simulink library "rtlsdr_book_library"  (R2014b)
settings: Solver=ode45  StartTime=0.0  StopTime=10.0  RelTol=1e-3
values from neighbouring files (symbols this model uses):
  frm = rmfield(frm , 'master_frame')    [image_frame_gen.m]    (also in import_rtlsdr_data.m = cast(frm,obj.data_type))
  src = rmfield(src , 'master_time')    [ASCII_frame_gen.m]
undefined symbols (not defined in the file or in its folder): den, dfilt, fdesignblkfcn, gcbh, iir, num, rtlsdr_frmsize, rtlsdr_fs
undefined symbols (not defined in the file): costas
libraries: dspsigops x6, commsynccomp2 x4, dspsrcs4 x2, dspstat3 x2, dspobslib x2, simulink_extras x2, dspmtrx3 x2, dsparch4 x1, rtlsdr_book_library x1, dspspect3 x1, commrflib2 x1
(part 1 of 5)
Description:
  | Software, Simulation Examples and Design Exercises Licence Agreement
  | 
  | This license agreement refers to the simulation examples, design exercises and files,
  | and associated software MATLAB and Simulink resources that accompany the book:
  | 
  |      Title: Software Defined Radio using MATLAB & Simulink and the RTL-SDR
  |      Published by Strathclyde Academic Media, 2015
  |      Authored by Robert W. Stewart, Kenneth W. Barlee, Dale S.W. Atkinson,
  |      and Louise H. Crockett
  | 
  | and made available as a download from, www.desktopSDR.com or variously acquired
  | by other means such as via USB storage, cloud storage, disk or any other electronic
  | or optical or magnetic storage mechanism. These files and associated software may
  | be used subject to the terms of agreement of the conditions below:
  | 
  |     Copyright © 2015 Robert W. Stewart, Kenneth W. Barlee, Dale S.W. Atkinson,
  |     and Louise H. Crockett
  |     All rights reserved.
  | 
  | Redistribution and use in source and binary forms, with or without modification, are
  | permitted provided that the following conditions are met:
  | 
  |    1.  Redistributions of source code must retain the above copyright notice, this list of
  |         conditions and the following disclaimer.
  | 
  |    2.  Redistributions in binary form must reproduce the above copyright notice, this
  |         list of conditions and the following disclaimer in the documentation and/or other
  |         materials provided with the distribution.
  | 
  |    3.  Neither the name of the copyright holder nor the names of its contributors may
  |         be used to endorse or promote products derived from this software without
  |         specific prior written permission.
  | 
  |    4.  In all cases, the software is, and all modifications and derivatives of the
  |         software shall be, licensed to you solely for use in conjunction with The
  |         MathWorks, Inc. products and service offerings.
  | 
  | THIS SOFTWARE IS PROVIDED BY THE COPYRIGHT HOLDERS AND CONTRIBUTORS
  | "AS IS" AND ANY EXPRESS OR IMPLIED WARRANTIES, INCLUDING, BUT NOT LIMITED
  | TO, THE IMPLIED WARRANTIES OF MERCHANTABILITY AND FITNESS FOR A
  | PARTICULAR PURPOSE ARE DISCLAIMED. IN NO EVENT SHALL THE COPYRIGHT
  | HOLDER OR CONTRIBUTORS BE LIABLE FOR ANY DIRECT, INDIRECT, INCIDENTAL,
  | SPECIAL, EXEMPLARY, OR CONSEQUENTIAL DAMAGES (INCLUDING, BUT NOT
  | LIMITED TO, PROCUREMENT OF SUBSTITUTE GOODS OR SERVICES; LOSS OF USE,
  | DATA, OR PROFITS; OR BUSINESS INTERRUPTION) HOWEVER CAUSED AND ON ANY
  | THEORY OF LIABILITY, WHETHER IN CONTRACT, STRICT LIABILITY, OR TORT
  | (INCLUDING NEGLIGENCE OR OTHERWISE) ARISING IN ANY WAY OUT OF THE USE
  | OF THIS SOFTWARE, EVEN IF ADVISED OF THE POSSIBILITY OF SUCH DAMAGE.
  | 
  | 
  | Audio Tracks used in Simulations Examples and Design Exercises
  | 
  | The music and vocal files used within the Examples files and software within the book
  | were variously written, arranged, performed, recorded and produced by Garrey Rice,
  | Adam Struth, Jamie Struth, Iain Thistlethwaite and also Marshall Craigmyle who
  | collectively, and individually where appropriate, assert and retain all of their copyright,
  | performance and artistic rights. Permission to use and reproduce this music is
  | granted for all purposes associated with MATLAB and Simulink software and the
  | simulation examples and design exercises files that accompany this book. Requests to
  | use the music for any other purpose should be directed to: info@desktopSDR.com.
  | For information on music track names, full credits, and links to the musicians please
  | refer to www.desktopSDR.com/more/audio.
settings Model: Creator=dkb10130  LastModifiedBy=ehb10152

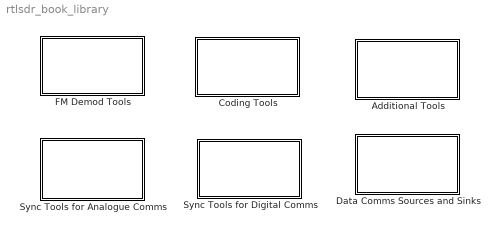
== system rtlsdr_book_library ==
  Additional Tools : Subsystem
      mask Display: disp('Additional\nTools');
  Coding Tools : Subsystem
      mask Display:
      | plot(-2,-2.5,...
      |      105,1.1,...
      |      [0  10 10.1 50 50.1 60 60.01 100],[0 0 1 1 0 0 1 1]); % bitstream
      | 
      | disp('\nCoding\nTools ');
  Data Comms Sources and Sinks : Subsystem
      mask Display:
      | plot(-2,-2.5,...
      |      105,1.1,...
      |      [45 45.01 50 50.01 55 55.01 60 60.01 65 65.01 70 70.01 75 75.01 80 80.01 85 85.01 90 90.01 95 95.01 100],...
      |      [0  1    1  0    0  0    0  1    1  0    0  1    1  1    1  0     0  1    1  0     0  1    1]); % bitstream
      | 
      | disp('\n010110                 \n\n\n\n')
      | disp('\nData Sources\nand Sinks');
  FM Demod Tools : Subsystem
      mask Display:
      | i = sin(2*pi*12*[0:0.001:0.4]);
      | fm = 2*sin(2*pi*80*[0:0.001:0.4] + cumsum(i)/3);
      | 
      | plot(-0.01,-13,...
      |     0.41,2.5,...
      |     [0:0.001:0.4], [fm(21:219), -2.5, 2.5, 2*i(202:end)]);
      | 
      | clear('i','fm');
      | 
      | disp('\nFM Demod\nTools');
  Sync Tools for Analogue Comms : Subsystem
      mask Display:
      | i = sin(2*pi*12*[0:0.001:0.4]);
      | am = sin(2*pi*99*[0:0.001:0.4]) .* (i+1.5);
      | 
      | plot(-0.01,-13,...
      |     0.41,2.5,...
      |     [0:0.001:0.4], [am(21:219), -2.5, 2.5, 2*i(202:end)]);
      | 
      | clear('i','am');
      | 
      | disp('\nSync Tools for\nAnalogue Comms');
  Sync Tools for Digital Comms : Subsystem
      mask Display:
      | plot(-2,-2.5,...
      |      125,1.1,...
      |      [5 15 15.1 30 30 45 45.1 60 60.1 75 75.1 90 90.1 105 105.1 115],[0.5 0.5 1 1 0.2 0.2 1 1 0.2 0.2 1 1 0.2 0.2 0.5 0.5]);  % Received Signal
      | 
      | plot(-2,-2.5,...
      |      125,1.1,...
      |      [5 11.5 11.6 27 27 42.5 42.6 58 58.1 73.5 73.6 89 89.1 104.5 104.6 115],[0.3,0.3,0.8,0.8,-0.1,-0.1,0.8,0.8,-0.1,-0.1,0.8,0.8,-0.1,-0.1,0.3,0.3]);  % Local Signal
      | 
      | disp('\nSync Tools for\nDigital Comms');

== system rtlsdr_book_library/Additional Tools ==
  433MHz Tuner Freq and Gain Control : Subsystem  mask{tuner_freq=433.0, tuner_gain=25}
      mask prompts: tuner_freq "Frequency (MHz)"; tuner_gain "Gain (dB)"
      mask DialogControl DescGroupVar Prompt: Tuner Frequency and Gain Control
      mask DialogControl DescTextVar Prompt: Use the control below to change the tuner frequency and gain.
  AM-SSB Modulator : Subsystem  mask{ac=1, phc=0, fc=40e3, fs=120e3, frm_size=1500}
      mask prompts: ac "Carrier Amplitude:"; phc "Carrier Phase (rads):"; fc "Carrier Frequency (Hz):"; fs "Sampling Frequency (Hz):"; frm_size "Output Frame Size:"
      mask DialogControl DescTextVar Prompt: This block AM-SSB modulates an information signal, outputting both the AM-SLSB and AM-SUSB variants. We have also output the carrier, which can be used as a reference.
  Import RTL-SDR Data : Subsystem  InitFcn=|  StopFcn=|  mask{filename=rtlsdr_data.mat, frm_size=4096, data_type=single}
      InitFcn=|
      | try
      |    load(get_param(gcb,'filename'));
      |    [nfrm,rtlsdr_frmsize] = size(rtlsdr_data.data);
      |    rtlsdr_fs = rtlsdr_frmsize/rtlsdr_data.TimeInfo.Increment;
      | catch
      |       error(['Unable to read file "',get_param(gcbh,'filename'),...
      |            '". No such file or directory. Please check that the filename',...
      |            ' you entered is correct, and contains the ".mat" extension.']);
      | end
      StopFcn=|
      | clear(...
      | 'rtlsdr_frmsize',...
      | 'rtlsdr_fs',...
      | 'nfrm',...
      | 'rtlsdr_data' );
      mask prompts: filename "File Name:"; frm_size "Output Frame Size:"; data_type "Output Data Type:"
      settings: CloseFcn=|
      | try
      |    load(get_param(gcb,'filename'));
      |    [nfrm,rtlsdr_frmsize] = size(rtlsdr_data.data);
      |    rtlsdr_fs = rtlsdr_frmsize/rtlsdr_data.TimeInfo.Increment;
      | catch
      |       error(['Unable to read file "',get_param(gcbh,'filename'),...
      |            '". No such file or directory. Please check that the filename',...
      |            ' you entered is correct, and contains the ".mat" extension.']);
      | end
      mask Callback filename:
      | set_param([gcb '/From File'], 'Filename',...
      |             get_param(gcbh,'filename'));
      mask TypeOptions data_type: int16 | single | double
      mask DialogControl Control2 Prompt: Browse
      mask DialogControl Control2 Callback:
      | % browse for file
      | [filename,path] = uigetfile({'*.mat'},'Select an RTL-SDR Data File');
      | 
      | % if in current folder, only use filename
      | if strcmp([pwd,filesep],path)
      | 
      |     try
      |         % try to set the filename in the box
      |         set_param(...
      |             gcb,...
      |             'filename',...
      |             filename );
      |         % try to import the data
      |         load(get_param(gcb,'filename'));
      |         rtlsdr_frmsize = length(rtlsdr_data.data);
      |         [nfrm,rtlsdr_frmsize] = size(rtlsdr_data.data);
      |         rtlsdr_fs = rtlsdr_frmsize/rtlsdr_data.TimeInfo.Increment;
      |     end
      | % else use full filepath
      | else
      | 
      |     try
      |         % try to set the filename in the box
      |         set_param(...
      |             gcb,...
      |             'filename',...
      |             [path,filename] );
      |         % try to import the data
      |      	load(get_param(gcb,'filename'));
      |         [nfrm,rtlsdr_frmsize] = size(rtlsdr_data.data);
      |         rtlsdr_fs = rtlsdr_frmsize/rtlsdr_data.TimeInfo.Increment;
      |     end
      | end
      | 
      | clear('path','filename');
      mask Display:
      | % try to apply icon
      | try
      |     root = which('rtlsdr_book_library');
      |     root = root(1:end-length('rtlsdr_book_library/rtlsdr_book_library.slx'));
      |     image([root,'rtlsdr_book_library/block_icons/icon__load_rtlsdr_data.png'],[0,0,125,60]);
      | end
      | 
      | % if file accessible
      | try
      |     load(get_param(gcb,'filename'));
      |         [nfrm,rtlsdr_frmsize] = size(rtlsdr_data.data);
      |         rtlsdr_fs = rtlsdr_frmsize/rtlsdr_data.TimeInfo.Increment;
      |         %rtlsdr_fs = 1/rtlsdr_data.TimeInfo.Increment;
      | 
      |     % convert to kHz
      |     fs = rtlsdr_fs/1000;
      | 
      |     % if MHz.. convert to MHz and display
      |     if fs > 999
      |         fs = fs/1000;
      |         fprintf(['\n\n\n               fs = ',num2str(fs),'MHz']);
      | 
      |     % else display kHz
      |     else
      |         fprintf(['\n\n\n              fs = ',num2str(fs),'kHz']);
      |     end
      | 
      | catch
      |     % display nothing
      |     fprintf('\n\n\n   fs = ');
      | end
  Model Information : Subsystem
  Remove DC Component : Subsystem
      mask DialogControl DescGroupVar Prompt: Remove DC Component
      mask DialogControl DescTextVar Prompt: This block removes the DC component of signals input to it.
  Save RTL-SDR Data : Subsystem  InitFcn=|  mask{file_name=rtlsdr_data.mat}
      | stop_time = get_param(gcs,'StopTime');
      | 
      | if str2num(stop_time) > 120
      | 
      |    dlg = warndlg(...
      |       ['Running this simulation for ',stop_time,' seconds will create a very large data file!'],...
      |       'Warning: Save RTL-SDR Data',...
      |       'modal');
      |    
      |    uiwait(dlg);
      | 
      | end
      | 
      | clear('stop_time');
      mask prompts: file_name "File Name:"
      mask Callback file_name:
      | set_param([gcb '/To File'], 'Filename',...
      |             get_param(gcbh,'file_name'))
      mask DialogControl Control3 Prompt: Browse
      mask DialogControl Control3 Callback:
      | % browse for file
      | [filename,path] = uiputfile({'*.mat'},'Create an RTL-SDR Data File');
      | 
      | % if in current folder, only use filename
      | if strcmp([pwd,filesep],path)
      | 
      |     % try to set the filename in the box
      |     try
      |         set_param(...
      |             gcb,...
      |             'file_name',...
      |             filename );
      |     end
      | % else use full filepath
      | else
      | 
      |     % try to set the filename in the box
      |     try
      |         set_param(...
      |             gcb,...
      |             'file_name',...
      |             [path,filename] );
      |     end
      | end
      | 
      | clear('path','filename');
      mask Display:
      | % try to apply icon
      | try
      |     root = which('rtlsdr_book_library');
      |     root = root(1:end-length('rtlsdr_book_library/rtlsdr_book_library.slx'));
      |     image([root,'rtlsdr_book_library/block_icons/icon__save_rtlsdr_data.png'],[0,0,125,60]);
      | end

== system rtlsdr_book_library/Coding Tools ==
  Differential QPSK Decoder : Subsystem  mask{op_buff_len=2}
      mask prompts: op_buff_len "Enter the required output frame size:"
      mask DialogControl DescGroupVar Prompt: Differential QPSK Decoder
      mask DialogControl DescTextVar Prompt: This subsystem contains the combinatorial logic required to implement a QPSK Decoder.
  Differential QPSK Encoder : Subsystem  mask{op_buff_len=2}
      mask prompts: op_buff_len "Enter the required output frame size:"
      mask DialogControl DescGroupVar Prompt: Differential QPSK Encoder
      mask DialogControl DescTextVar Prompt: This subsystem contains the combinatorial logic required to implement a QPSK Encoder.

== system rtlsdr_book_library/Data Comms Sources and Sinks ==
  "  ASCII Transfer Binary Source" : Subsystem  mask(Bit Source Generator - Numbered Frames){msg_tx=Hello World!, fs=2e3, ascii_len=8}
      mask prompts: msg_tx "Message String:"; fs "Bitrate (Sampling Frequency):"; ascii_len "ASCII Character Bit Length:"
      mask help: The block converts ASCII characters from the 'Message String' field to ASCII bits. This then forms the payload of an individual frame and is appended to the preamble sequence, which forms the header. The output of this block is a data frame of bits that will be modulated and transmitted.
      mask init:
      | try
      |     ASCII_frame_gen;
      | catch ME
      |     if(strcmp(ME.identifier,'MATLAB:UndefinedFunction'))
      |         error('Unable to find "ASCII_frame_gen.m".');
      |     end
      |     rethrow(ME);
      | end
      settings: ModelCloseFcn=clear('msg_output','rec','run_time','src')
      mask Callback msg_tx: ASCII_frame_gen;
      mask Callback fs: ASCII_frame_gen;
      mask Callback ascii_len: ASCII_frame_gen;
      mask Display:
      | try
      |     ASCII_frame_gen;
      | catch ME
      |     if(strcmp(ME.identifier,'MATLAB:UndefinedFunction'))
      |         error('Unable to find "ASCII_frame_gen.m".');
      |     end
      |     rethrow(ME);
      | end
      | 
      | %% FOR MASK
      | % number of chars in message
      | src.num_chars = src.len(:,1);
      | % create text string
      | icon_text = ['Bit Source - Numbered Frames\n\n'...
      |              'Message Length (chars) = ',num2str(src.num_chars),'\n\n'...
      |              'Frame Size (bits) = ',num2str(src.master_frame_len)];
      | % display on block
      | disp(icon_text);
  ASCII Decoding : Subsystem  mask(ASCII Reconstruction){msg_len=16, ascii_len=8}
      mask prompts: msg_len "Message Length (chars):"; ascii_len "ASCII Character Bit Length:"
      mask help: The block reconstructs the ASCII strings from the input payload.
  Image Reconstruction : Subsystem  InitFcn=|  mask(Image Reconstruction){}
      | % create figure window, plot empty image then hide
      | hfig = figure;
      | imshow(uint8(zeros(100,100)),'InitialMagnification',250);
      | hfig.Visible = 'off';
      mask help: This block will receive and process frames of image data. When the full image has been receieved, the simulation will pause, and the image will be displayed.
      settings: CloseFcn=clear('hfig','hax');
      settings: PauseFcn=|
      | % set current figure to handle
      | set(0,'CurrentFigure',hfig);
      | 
      | % make plot visible if not already
      | hfig.Visible = 'on'
      | 
      | % plot image
      | imshow(uint8(image),'InitialMagnification',250);
      | 
      | % configure image figure window
      | hfig.MenuBar = 'none';
      | hfig.ToolBar = 'none';
      | hfig.Resize = 'off';
      | hfig.Name = 'Received Image';
      | hfig.NumberTitle = 'off';
      | hfig.Position = [hfig.Position(1)+45,hfig.Position(2)+3,330,335];
      | hax = gca;
      | hax.Units = 'pixels';
      | hax.Position = [40,45,250,250];
      | 
      | % resume simulation
      | set_param(bdroot, 'SimulationCommand', 'continue')
  Image Transfer Binary Source : Subsystem  mask(Bit Source Generator - Image Transfer){filename=image1.mat, fs=2e3, binary_len=8}
      mask prompts: filename "Image Filename:"; fs "Bitrate (Sampling Frequency):"; binary_len "Image Pixel Bit Depth:"
      mask help: The block allows the user to enter the filename of an image that they wish to transmit. It converts the image's pixels from decimal values to binary bit representations, and generates the number of frames required to transfer the data to the receiver. Each frame's header has a preamble and a number of fields that contain information about the frame, to support the recovery of the data at the receiver. The remaining space in each frame is then dedicated to the payload, which contains a part of the total data to be transferred.
      mask init:
      | try
      |     image_frame_gen;
      | catch ME
      |     switch ME.identifier
      |         case 'MATLAB:load:couldNotReadFile'
      |             error(['Unable to locate "', get_param(gcb,'filename'),'". Please check that the image filename is correct.']);
      |         case 'MATLAB:UndefinedFunction'
      |             error('Unable to find "image_frame_gen.m".');
      |         otherwise
      |             rethrow(ME)
      |     end
      | end
      settings: ModelCloseFcn=clear('frm')
      mask Callback filename:
      | %% PULL DATA FROM MASK
      | frm.filename = get_param(gcbh,'filename');
      | 
      | set_param(gcb,'filename',frm.filename)
      | 
      | try
      |     image_frame_gen;
      | catch ME
      |     switch ME.identifier
      |         case 'MATLAB:load:couldNotReadFile'
      |             error(['Unable to locate "', get_param(gcb,'filename'),'". Please check that the image filename is correct.']);
      |         case 'MATLAB:UndefinedFunction'
      |             error('Unable to find "image_frame_gen.m".');
      |         otherwise
      |             rethrow(ME)
      |     end
      | end
      mask Callback fs:
      | %% PULL DATA FROM MASK
      | frm.fs = str2num(get_param(gcbh,'fs'));
      mask Callback binary_len:
      | %% PULL DATA FROM MASK
      | frm.binary_len = str2num(get_param(gcbh,'binary_len'));
      mask DialogControl Control2 Prompt: Browse
      mask DialogControl Control2 Callback:
      | % root to library folder
      | rootlib = which('rtlsdr_book_library');
      | rootlib = rootlib(1:end-length('/rtlsdr_book_library.slx'));
      | 
      | % browse for file
      | [filename,path] = uigetfile({[rootlib,'/*.mat']},'Select a MAT image file');
      | 
      | % if in current folder, only use filename
      | if strcmp([rootlib,filesep],path)
      | 
      |     try
      |         % try to set the filename in the box
      |         set_param(...
      |             gcb,...
      |             'filename',...
      |             filename);
      |         % try to import the data
      |         load(get_param(gcb,'filename'));
      |     end
      | % else use full filepath
      | else
      | 
      |     try
      |         % try to set the filename in the box
      |         set_param(...
      |             gcb,...
      |             'filename',...
      |             [path,filename] );
      |         % try to import the data
      |      	load(get_param(gcb,'filename'));
      |     end
      | end
      | 
      | clear('path','filename');
      mask Display:
      | try
      |     image_frame_gen;
      | catch ME
      |     switch ME.identifier
      |         case 'MATLAB:load:couldNotReadFile'
      |             error(['Unable to locate "', get_param(gcb,'filename'),'". Please check that the image filename is correct.']);
      |         case 'MATLAB:UndefinedFunction'
      |             error('Unable to find "image_frame_gen.m".');
      |         otherwise
      |             rethrow(ME)
      |     end
      | end
      | 
      | %% FOR MASK
      | try
      |     % create text string
      |     blk_text = ['Bit Source - Image Transfer\n\n',...
      |                 'Dimensions (pixels) = ',num2str(frm.image_size(:,1)),' x ',num2str(frm.image_size(:,2)),'\n\n'...
      |                 'Frame Size (bits) = ',num2str(frm.frame_len)];
      |     % display on block
      |     disp(blk_text);
      | catch
      |     % create error text string
      |     error_text = ['Unable to load image -\n\n',...
      |                   'Check image filename and MATLAB \ndirectory are set correctly.'];
      |     %display warning if image cannot be loaded
      |     disp(error_text);
      | end

== system rtlsdr_book_library/FM Demod Tools ==
  FM De-emphasis Filter : Subsystem  mask{region=Europe, Asia, fs=48e3}
      mask prompts: region "Filter Region"; fs "Sampling Frequency (Hz)"
      mask init:
      | deemp.fs = 48e3;
      | deemp.region_sw = 1;
      | 
      | [deemp.num_eu,deemp.den_eu] = butter(1,3183.1/(deemp.fs/2));
      | [deemp.num_us,deemp.den_us] = butter(1,2122.1/(deemp.fs/2));
      settings: ModelCloseFcn=clear('deemp')
      mask TypeOptions region: Europe, Asia | USA
      mask Callback region:
      | deemp.fs = str2num( get_param(gcbh, 'fs') );                    % sampling frequnecy
      | deemp.radio_button = get_param(gcbh, 'region');                 % current radio button string
      | 
      | [deemp.num_eu,deemp.den_eu] = butter(1,3183.1/(deemp.fs/2));    % calculate filter weights for both modes
      | [deemp.num_us,deemp.den_us] = butter(1,2122.1/(deemp.fs/2));
      | 
      | switch deemp.radio_button                                       % convert radio button string to number
      |     case 'Europe, Asia'                                         % (used to control multiport switch)
      |         deemp.region_sw = 1;
      |     case 'USA'
      |         deemp.region_sw = 2;
      |     otherwise
      |         error('Invalid region selected');
      | end
      mask Callback fs:
      | deemp.fs = str2num( get_param(gcbh, 'fs') );                    % sampling frequnecy
      | deemp.radio_button = get_param(gcbh, 'region');                 % current radio button string
      | 
      | [deemp.num_eu,deemp.den_eu] = butter(1,3183.1/(deemp.fs/2));    % calculate filter weights for both modes
      | [deemp.num_us,deemp.den_us] = butter(1,2122.1/(deemp.fs/2));
      | 
      | switch deemp.radio_button                                       % convert radio button string to number
      |     case 'Europe, Asia'                                         % (used to control multiport switch)
      |         deemp.region_sw = 1;
      |     case 'USA'
      |         deemp.region_sw = 2;
      |     otherwise
      |         error('Invalid region selected');
      | end
      mask DialogControl button Prompt: View Frequency Response
      mask DialogControl button Callback:
      | deemp.fs = str2num( get_param(gcbh, 'fs') );                    % sampling frequnecy
      | deemp.radio_button = get_param(gcbh, 'region');                 % current radio button string
      | 
      | [deemp.num_eu,deemp.den_eu] = butter(1,3183.1/(deemp.fs/2));    % calculate filter weights for both modes
      | [deemp.num_us,deemp.den_us] = butter(1,2122.1/(deemp.fs/2));
      | 
      | switch deemp.radio_button                                       % convert radio button string to number
      |     case 'Europe, Asia'                                         % (used to control multiport switch)
      |         deemp.region_sw = 1;
      |     case 'USA'
      |         deemp.region_sw = 2;
      |     otherwise
      |         error('Invalid region selected');
      | end
      | 
      | if deemp.region_sw == 1                                         % run fvtool function
      |     deemp.h_fvtool =  fvtool(deemp.num_eu,deemp.den_eu,'fs',deemp.fs,'legend','on');
      |     legend(deemp.h_fvtool,'FM Deemphasis Filter Freq Response (EU, Asia)');
      | 
      | elseif deemp.region_sw == 2                                     % run fvtool function
      |     deemp.h_fvtool =  fvtool(deemp.num_us,deemp.den_us,'fs',deemp.fs,'legend','on');
      |     legend(deemp.h_fvtool,'FM Deemphasis Filter Freq Response (USA)');
      | end
      mask Display:
      | port_label('input', 1, 'sig_in')
      | port_label('output', 1, 'filt_out')
      | 
      | deemp.radio_button = get_param(gcbh, 'region');                 % current radio button string
      | 
      | switch deemp.radio_button                                       % convert radio button string to number
      |     case 'Europe, Asia'                                         % (used to control multiport switch)
      |         fprintf('Mode:\nEU + Asia');
      |     case 'USA'
      |         fprintf('Mode:\nUSA');
      |     otherwise
      |         error('Mask error - Invalid region selected');
      | end
  FM MPX Demultiplexer : Subsystem  InitFcn=|  mask{fs=120e3, fq=19e3, Kpd=3, Kphe=2, frm_size=4000}
      | % get fs
      | fs = str2num(get_param(gcb,'fs'));
      | 
      | % get fq
      | fq = str2num(get_param(gcb,'fq'));
      mask prompts: fs "Sampling Frequency (Hz):"; fq "Quiescent Frequency"; Kpd "Phase Detector Gain:"; Kphe "Phase Error Gain:"; frm_size "Output Frame Size:"
      mask init:
      | % get fs
      | fs = str2num(get_param(gcb,'fs'));
      | 
      | % get fq
      | fq = str2num(get_param(gcb,'fq'));
      | 
      | % peak notch design
      | fdesignblkfcn(get_param([gcb,'/Peak-Notch Filter'],'handle'), {'InitFcn'});
      | 
      | % iir design
      | [iir.b, iir.a] = cheby2(22,100,18e3/(fs/2),'low');
      | 
      | % nco design
      | nco.deltaf = 0.05;                              % nco freq resolution in Hz
      | nco.acc_wl = ceil(log2(1/((1/fs)*nco.deltaf))); % calc required wordlength
      | nco.sfdr = 80;                                  % spurious free dynamic range of nco (noise floor level)
      | nco.acc_quant = ceil((nco.sfdr-12)/6);          % calc number of quantised accumulator bits
      | nco.dither = ceil(nco.acc_wl - nco.acc_quant);  % calc nco dither
      | nco.op_wl = 10;                                 % set op word length
      | nco.op_frac = 8;                                % set op fractional bits
  FM Tuner Freq and Gain Control : Subsystem  mask{tuner_freq=100.0, tuner_gain=25}
      mask prompts: tuner_freq "Frequency (MHz)"; tuner_gain "Gain (dB)"
      mask DialogControl DescGroupVar Prompt: Tuner Frequency and Gain Control
      mask DialogControl DescTextVar Prompt: Use the control below to change the tuner frequency and gain.

== system rtlsdr_book_library/Sync Tools for Analogue Comms ==
  Costas Loop Demodulator : Subsystem  InitFcn=|  mask(Costas Loop){filter_type=Type 2, K1_param=(4*d*Bn*1/fs)/(Ko*Kp*(d+1/(4*d))), K2_param=(4*(Bn*1/fs)^2)/(Ko*Kp*(d+1/4*d)^2), fs=240e3, fq=40e3, Bn=1e3, d=0.707, frm_size=4096}
      | % get fs
      | fs = str2num(get_param(gcb,'fs'));
      mask prompts: filter_type "Loop Filter Type:"; K1_param "K1 (proportional path) :"; K2_param "K2 (integral path) :"; fs "Sampling Frequency (Hz):"; fq "Quiescent Frequency (Hz):"; Bn "Noise Bandwidth (Hz):"; d "Damping Ratio:"; frm_size "Output Frame Size:"
      mask help: Ensure you set the sampling frequency parameter to match the sampling frequency of the input signal, otherwise the loop will not function correctly.
      mask init:
      | % ------- synch loop design -------- %
      | A = 1;      % assume amplitude of input to PD is 1
      | Kp = A/2;   % phase detector is a multiplier 
      | Ko = 1;     % gain of NCO (normalised to fs)
      settings: ModelCloseFcn=clear('costas')
      mask TypeOptions filter_type: Type 1 | Type 2
      mask Callback filter_type:
      | % sync loop params needed for loop filter
      | A = 1;       % assume amplitude of input to PD is 1
      | Kp = A/2;    % phase detector is a multiplier
      | Ko = 1;      % gain of NCO (normalised to fs)
      | fs = str2num(get_param(gcb,'fs'));
      | fq = str2num(get_param(gcb,'fq'));
      | Bn = str2num(get_param(gcb,'Bn'));
      | d = str2num(get_param(gcb,'d'));
      | 
      | % get type - 1, 2 or 3
      | filter_type = get_param(gcb,'filter_type');
      | 
      | % if type 1, disable K2
      | if filter_type == 'Type 1'
      |     set_param(gcb,'K1_param','1');
      |     set_param(gcb,'K2_param','0');
      | end
      | 
      | % if type 2, enable K3
      | if filter_type == 'Type 2'
      |     set_param(gcb,'K1_param','(4*d*Bn*1/fs)/(Ko*Kp*(d+1/(4*d)))');
      |     set_param(gcb,'K2_param','(4*(Bn*1/fs)^2)/(Ko*Kp*(d+1/4*d)^2)');
      | end
      | 
      | % update coefficients
      | try
      |     costas.K1 = eval(get_param(gcb,'K1_param'));
      |     costas.K2 = eval(get_param(gcb,'K2_param'));
      | end
      | 
      | clear('A','Kp','Ko','fs','fq','Bn','d','filter_type');
  Phase Locked Loop Demodulator : Subsystem  StopFcn=clear('pll');  mask{filter_type=Type 2, K1_param=(4*d*Bn*1/fs)/(Ko*Kp*(d+1/(4*d))), K2_param=(4*(Bn*1/fs)^2)/(Ko*Kp*(d+1/4*d)^2), fs=240e3, fq=40e3, Bn=1e3, d=0.707, frm_size=4096}
      mask prompts: filter_type "Loop Filter Type:"; K1_param "K1 (proportional path) :"; K2_param "K2 (integral path) :"; fs "Sampling Frequency (Hz):"; fq "Quiescent Frequency (Hz):"; Bn "Noise Bandwidth (Hz):"; d "Damping Ratio:"; frm_size "Output Frame Size:"
      mask init:
      | % ------- synch loop design -------- %
      | A = 1;       % assume amplitude of input to PD is 1
      | Kp = A/2;    % phase detector is a multiplier
      | Ko = 1;      % gain of NCO (normalised to fs)
      | 
      | % update coefficients
      | try
      |     pll.K1 = eval(get_param(gcb,'K1_param'));
      |     pll.K2 = eval(get_param(gcb,'K2_param'));
      | end
      | 
      | set_param(gcb,'MaskEnables',{'on';'off';'off';  'on';'on';'on';'on';'on';});
      settings: ModelCloseFcn=clear('pll')
      mask TypeOptions filter_type: Type 1 | Type 2
      mask Callback filter_type:
      | % sync loop params needed for loop filter
      | A = 1;       % assume amplitude of input to PD is 1
      | Kp = A/2;    % phase detector is a multiplier
      | Ko = 1;      % gain of NCO (normalised to fs)
      | fs = str2num(get_param(gcb,'fs'));
      | fq = str2num(get_param(gcb,'fq'));
      | Bn = str2num(get_param(gcb,'Bn'));
      | d = str2num(get_param(gcb,'d'));
      | 
      | % get type - 1, 2 or 3
      | filter_type = get_param(gcb,'filter_type');
      | 
      | % if type 1, disable K2
      | if filter_type == 'Type 1'
      |     set_param(gcb,'K1_param','1');
      |     set_param(gcb,'K2_param','0');
      | end
      | 
      | % if type 2, enable K3
      | if filter_type == 'Type 2'
      |     set_param(gcb,'K1_param','(4*d*Bn*1/fs)/(Ko*Kp*(d+1/(4*d)))');
      |     set_param(gcb,'K2_param','(4*(Bn*1/fs)^2)/(Ko*Kp*(d+1/4*d)^2)');
      | end
      | 
      | % update coefficients
      | try
      |     pll.K1 = eval(get_param(gcb,'K1_param'));
      |     pll.K2 = eval(get_param(gcb,'K2_param'));
      | end
      | 
      | clear('A','Kp','Ko','fs','fq','Bn','d','filter_type');
      mask DialogControl Control3 Prompt: Ensure you set the sampling frequency parameter to match the sampling frequency of the input signal, otherwise the loop will not function correctly.

== system rtlsdr_book_library/Sync Tools for Digital Comms ==
  Coarse Freq Correction : Subsystem  mask(Coarse Frequency Correction){frm_size=4096}
      mask prompts: frm_size "Output Frame Size:"
      mask help: This block can be used to correct a frequency tuning offset. Because of the algorithm used, it works best when the input signal is at a low sampling rate.

== system rtlsdr_book_library/Additional Tools/433MHz Tuner Freq and Gain Control ==
  Constant1 : Constant
  Freq : Gain  Gain=tuner_freq
  Gain : Gain  Gain=tuner_gain
  MHz : Constant  Value=1e6
  freq_out : Outport
  gain_out : Outport  Port=2
  wires:
  Constant1/1 -> Gain/1
  Freq/1 -> freq_out/1
  Gain/1 -> gain_out/1
  MHz/1 -> Freq/1

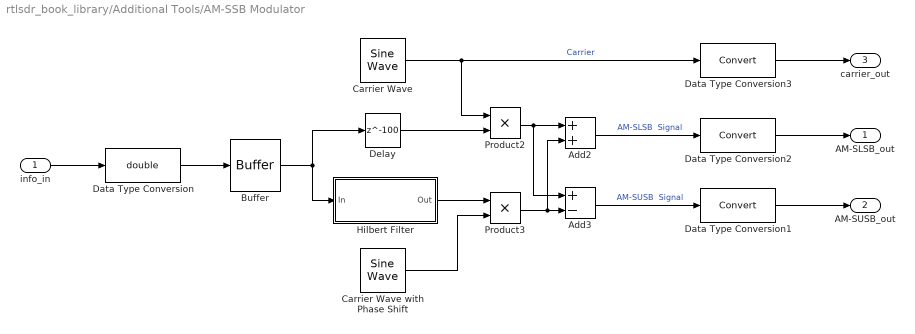
== system rtlsdr_book_library/Additional Tools/AM-SSB Modulator ==
  info_in : Inport
  Add2 : Sum
  Add3 : Sum  Inputs=+-
  Buffer : Buffer  N=frm_size  TreatMby1Signals=One channel
  Carrier Wave : dspsrcs4/Sine Wave  Amplitude=ac  Frequency=fc  Phase=phc  SampleMode=Discrete  OutComplex=Real  CompMethod=Trigonometric fcn  TableSize=Speed  SampleTime=1/fs  SamplesPerFrame=frm_size  ResetState=Restart at time zero  dataType=Inherit via back propagation  wordLen=16  udDataType=sfix(16)  fracBitsMode=Best precision  numFracBits=15  OutDataTypeStr=Inherit: Inherit via back propagation  LastOutDataTypeStr=Inherit: Inherit via back propagation
  Carrier Wave with Phase Shift : dspsrcs4/Sine Wave  Amplitude=ac  Frequency=fc  Phase=phc-pi/2  SampleMode=Discrete  OutComplex=Real  CompMethod=Trigonometric fcn  TableSize=Speed  SampleTime=1/fs  SamplesPerFrame=frm_size  ResetState=Restart at time zero  dataType=Inherit via back propagation  wordLen=16  udDataType=sfix(16)  fracBitsMode=Best precision  numFracBits=15  OutDataTypeStr=Inherit: Inherit via back propagation  LastOutDataTypeStr=Inherit: Inherit via back propagation
  Data Type Conversion : DataTypeConversion  OutDataTypeStr=double
  Data Type Conversion1 : DataTypeConversion
  Data Type Conversion2 : DataTypeConversion
  Data Type Conversion3 : DataTypeConversion
  Delay : Delay  DelayLength=100  InitialCondition=0  InputProcessing=Columns as channels (frame based)
  Hilbert Filter : Subsystem  DialogController=fdesignblkfcn  InitFcn=fdesignblkfcn(gcbh, {'InitFcn'});  mask(Hilbert Filter){}
      mask help: Design a Hilbert filter
      settings: CopyFcn=fdesignblkfcn(gcbh, {'CopyFcn'});
      mask Help: helpview(mapfilelocation('dsp'), 'dsphilbertfilter');
      mask Display: disp('Hilbert')
  Product2 : Product
  Product3 : Product
  AM-SLSB_out : Outport
  AM-SUSB_out : Outport  Port=2
  carrier_out : Outport  Port=3
  wires:
  Carrier Wave/1 -> Product2/1, Data Type Conversion3/1  "Carrier"
  Carrier Wave with Phase Shift/1 -> Product3/2
  Product2/1 -> Add3/1, Add2/1
  Product3/1 -> Add3/2, Add2/2
  Add2/1 -> Data Type Conversion2/1  "AM-SLSB  Signal"
  Add3/1 -> Data Type Conversion1/1  "AM-SUSB  Signal"
  Delay/1 -> Product2/2
  Hilbert Filter/1(Out) -> Product3/1
  Data Type Conversion/1 -> Buffer/1
  Buffer/1 -> Delay/1, Hilbert Filter/1(In)
  info_in/1 -> Data Type Conversion/1
  Data Type Conversion1/1 -> AM-SUSB_out/1
  Data Type Conversion2/1 -> AM-SLSB_out/1
  Data Type Conversion3/1 -> carrier_out/1

== system rtlsdr_book_library/Additional Tools/Import RTL-SDR Data ==
  note: outputs 1D arrays with length
      | matching the recording length
  note: resize 1D array
      | to user specified length
  note: convert 2D [usrlen x 1]
      | matrix to 1D array to match
      | RTL-SDR Receiver block
  Buffer : Buffer  N=frm_size  TreatMby1Signals=One channel
  Data Type Conversion : DataTypeConversion  OutDataTypeStr=data_type
  From File : FromFile  FileName=rtlsdr_data.mat  SampleTime=rtlsdr_frmsize/rtlsdr_fs  ExtrapolationAfterLastDataPoint=Ground value
  Reshape : Reshape
  data_out : Outport
  wires:
  From File/1 -> Data Type Conversion/1
  Data Type Conversion/1 -> Buffer/1
  Buffer/1 -> Reshape/1
  Reshape/1 -> data_out/1
